simulink model "SMC_LAB"  (R2020a)
settings: Solver=VariableStepAuto  StartTime=0.0  StopTime=10  RelTol=1e-3
settings Model: Creator=USER  LastModifiedBy=User Account

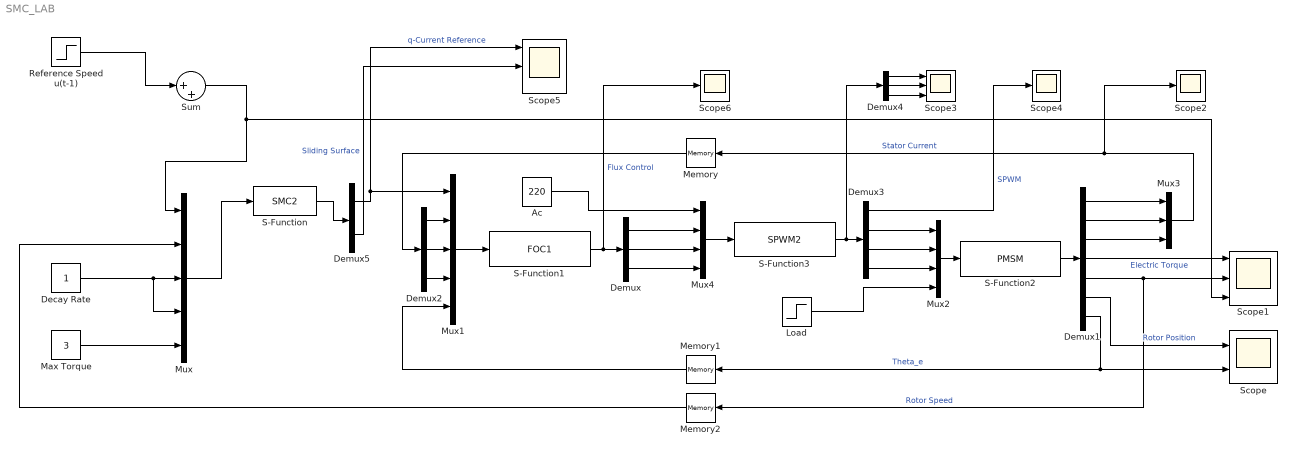
== system SMC_LAB ==
  Ac : Constant  Value=220
  Decay Rate : Constant
  Demux : Demux  Outputs=3
  Demux1 : Demux  Outputs=7
  Demux2 : Demux  Outputs=3
  Demux3 : Demux
  Demux4 : Demux  Outputs=3
  Demux5 : Demux  Outputs=2
  Load : Step  Time=5  After=5  SampleTime=0
  Max Torque : Constant  Value=3
  Memory : Memory
  Memory1 : Memory
  Memory2 : Memory
  Mux : Mux  Inputs=5
  Mux1 : Mux  Inputs=5
  Mux2 : Mux
  Mux3 : Mux  Inputs=3
  Mux4 : Mux
  Reference Speed u(t-1) : Step  After=20  SampleTime=0
  S-Function : S-Function  FunctionName=SMC2  SFunctionDeploymentMode=off  EnableBusSupport=off
  S-Function1 : S-Function  FunctionName=FOC1  SFunctionDeploymentMode=off  EnableBusSupport=off
  S-Function2 : S-Function  FunctionName=PMSM  SFunctionDeploymentMode=off  EnableBusSupport=off
  S-Function3 : S-Function  FunctionName=SPWM2  SFunctionDeploymentMode=off  EnableBusSupport=off
  Scope : Scope  NumInputPorts=2
  Scope1 : Scope  NumInputPorts=3
  Scope2 : Scope
  Scope3 : Scope  NumInputPorts=3
  Scope4 : Scope
  Scope5 : Scope  NumInputPorts=3
  Scope6 : Scope
  Sum : Sum  Inputs=|++
  wires:
  Demux5/2 -> Scope5/2  "Sliding Surface"
  Demux3/2 -> Mux2/1
  S-Function3/1 -> Demux4/1, Demux3/1
  Demux/2 -> Mux4/3
  Memory1/1 -> Mux1/5
  Memory/1 -> Demux2/1
  Memory2/1 -> Mux/2
  Demux4/2 -> Scope3/2
  Demux4/3 -> Scope3/3
  Mux4/1 -> S-Function3/1
  S-Function2/1 -> Demux1/1
  Demux3/3 -> Mux2/2
  Demux2/1 -> Mux1/2
  Demux/1 -> Mux4/2
  Demux1/6 -> Scope/1  "Rotor Position"
  Demux3/1 -> Scope4/1  "SPWM"
  Demux/3 -> Mux4/4
  Reference Speed u(t-1)/1 -> Sum/1
  Demux2/3 -> Mux1/4
  Demux1/7 -> Memory1/1, Scope/2  "Theta_e"
  Ac/1 -> Mux4/1
  Demux4/1 -> Scope3/1
  Mux1/1 -> S-Function1/1
  Demux1/4 -> Scope1/1  "Electric Torque"
  Demux5/1 -> Scope5/1, Mux1/1  "q-Current Reference"
  Demux1/5 -> Memory2/1, Scope1/2  "Rotor Speed"
  Mux3/1 -> Memory/1, Scope2/1  "Stator Current"
  Demux1/2 -> Mux3/2
  Demux2/2 -> Mux1/3
  Demux3/4 -> Mux2/3
  Demux1/1 -> Mux3/1
  S-Function/1 -> Demux5/1
  Demux1/3 -> Mux3/3
  Mux2/1 -> S-Function2/1
  S-Function1/1 -> Scope6/1, Demux/1  "Flux Control"
  Mux/1 -> S-Function/1
  Decay Rate/1 -> Mux/4, Mux/3
  Max Torque/1 -> Mux/5
  Load/1 -> Mux2/4
  Sum/1 -> Mux/1, Scope1/3
